simulink model "DCACmotor08022311"  (R2022b)
settings: Solver=VariableStepDiscrete  StartTime=0.0  StopTime=0.5  MaxStep=1e-4  RelTol=1e-3
libraries: spsVoltageMeasurementLib x9, spsSeriesRLCBranchLib x3, spsGroundLib x2, spsDCVoltageSourceLib x1, spsAsynchronousMachinepuUnitsLib x1, spsOnDelayLib x1, simulink x1, spsThreePhaseProgrammableVoltageSourceLib x1, spsUniversalBridgeLib x1, spsCurrentMeasurementLib x1, spspowerguiLib x1
settings Model: Creator=Lenovo  LastModifiedBy=ASUS
settings SolverCC: AlgebraicLoopSolver=TrustRegion
settings DataIOCC: ReturnWorkspaceOutputs=off
settings DebuggingCC: UnconnectedInputMsg=warning  UnconnectedOutputMsg=warning  UnconnectedLineMsg=warning  SFMachineParentedDataDiag=warning  ArithmeticOperatorsInVariantConditions=warning
settings ModelReferenceCC: EnableRefExpFcnMdlSchedulingChecks=on
settings SFSimCC: SimUseLocalCustomCode=off  CustomCodeUndefinedFunction=UseInterfaceOnly
settings RTWCC: RTWUseLocalCustomCode=off  DLArmComputeVersion=19.05

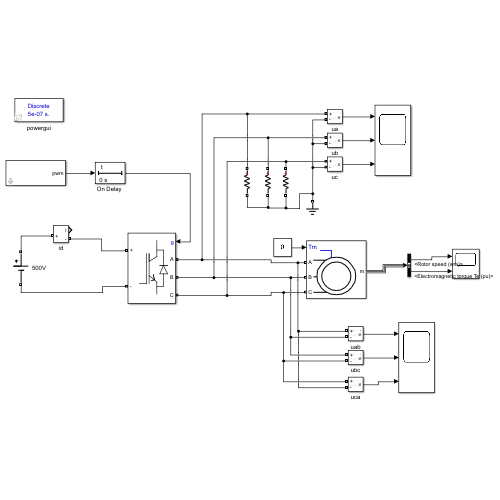
[thumbnail: Simulink's stored preview of the top-level diagram]
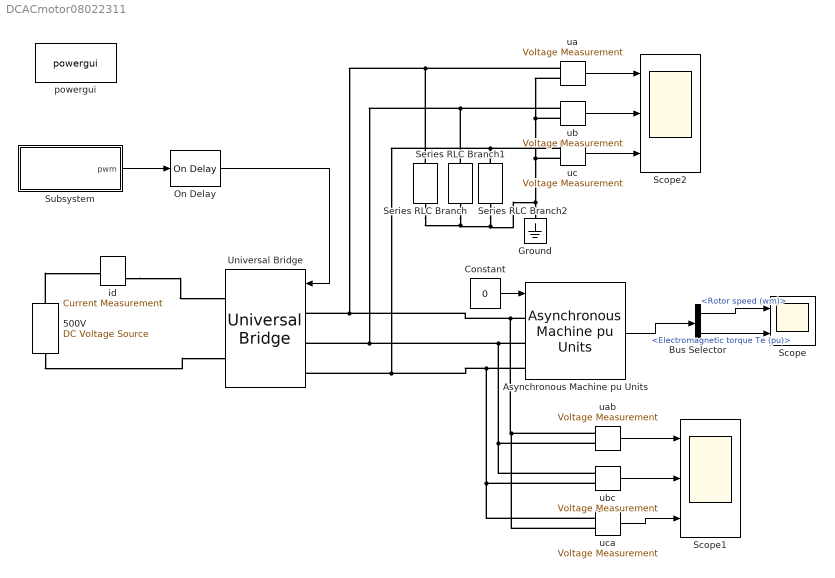
== system DCACmotor08022311 ==
  500V : spsDCVoltageSourceLib/DC Voltage Source  Amplitude=500  Measurements=None
  Asynchronous Machine pu Units : spsAsynchronousMachinepuUnitsLib/Asynchronous Machine pu Units  RotorType=Squirrel-cage  PresetModel=No  MechanicalLoad=Torque Tm  ShowDetailedParameters=on  ReferenceFrame=Rotor  Units=pu  MeasurementBus=off  NominalParameters=[3730 460 60]  VoltageRatio=1  Stator=[0.01965 0.0397]  Rotor=[0.01909 0.0397]  Cage1=[0.01909 0.0397]  Cage2=[0.01909 0.0397]  Lm=1.354  Mechanical=[0.09526 0.05479 2]  PolePairs=2  InitialConditions="[ 1,0   0,0,0   0,0,0 ]"  SimulateSaturation=off  Saturation="[0.212,0.4201,0.8125,1.0979,1.4799,2.2457,3.2586,4.5763,6.4763 ;   0.5,0.7,0.9,1,1.1,1.2 ,1.3,1.4,1.5]"  LoadFlowParameters=0  TsPowergui=0  TsBlock=-1  IterativeModel=Trapezoidal non iterative  IterativeDiscreteModel=Trapezoidal non iterative  Pmec=0
      settings: LibrarySourceBlock=|
      | sps_lib/Electrical Machines/Asynchronous Machine
      | pu Units
  Bus Selector : BusSelector  OutputSignals=Mechanical.Rotor speed (wm),Mechanical.Electromagnetic torque Te (pu)
  Constant : Constant  Value=0
  Ground : spsGroundLib/Ground  LConnTagsString=a
  "On Delay " : spsOnDelayLib/On Delay  DelayType=On delay  delay=0  ic=0  Ts=0
  Scope : Scope  NumInputPorts=2
  Scope1 : Scope  NumInputPorts=3
  Scope2 : Scope  NumInputPorts=3
  Series RLC Branch : spsSeriesRLCBranchLib/Series RLC Branch  LConnTagsString=__new0  RConnTagsString=__new0  BranchType=R  Resistance=1  Inductance=1e-3  SetiL0=off  InitialCurrent=0  Capacitance=1e-6  Setx0=off  InitialVoltage=0  Measurements=None
  Series RLC Branch1 : spsSeriesRLCBranchLib/Series RLC Branch  LConnTagsString=__new0  RConnTagsString=__new0  BranchType=R  Resistance=1  Inductance=1e-3  SetiL0=off  InitialCurrent=0  Capacitance=1e-6  Setx0=off  InitialVoltage=0  Measurements=None
  Series RLC Branch2 : spsSeriesRLCBranchLib/Series RLC Branch  LConnTagsString=__new0  RConnTagsString=__new0  BranchType=R  Resistance=1  Inductance=1e-3  SetiL0=off  InitialCurrent=0  Capacitance=1e-6  Setx0=off  InitialVoltage=0  Measurements=None
  Subsystem : Subsystem  mask{m=1, fc=1500, f=50}
      mask prompts: m "m(0<m<=1)"
  Universal Bridge : spsUniversalBridgeLib/Universal Bridge  Arms=3  SnubberResistance=1e5  SnubberCapacitance=inf  Device=IGBT / Diodes  Ron=1e-3  Lon=0  ForwardVoltages="[  0  0  ]"  ForwardVoltage=0  GTOparameters=[ 10e-6 , 20e-6 ]  IGBTparameters=[ 1e-6 , 2e-6 ]  Measurements=None  Measurements_2=None  converterType=Rectifier
  id : spsCurrentMeasurementLib/Current Measurement  PhasorSimulation=off  OutputType=Complex  PSBequivalent=0
  powergui : spspowerguiLib/powergui  Priority=1  SimulationMode=Discrete  SampleTime=5e-7  frequency=60  Iterations=50  frequencyindice=60  Pbase=100e6  ErrMax=1e-4  UnitsV=kV  UnitsW=MW  buscounter=0  FunctionMessages=off  echomessages=off  EnableUseOfTLC=off  CurrentSourceSwitches=off  DisableSnubberDevices=off  DisableRonSwitches=off  DisableVfSwitches=off  DisplayEquations=off  AutomaticDiscreteSolvers=off  SolverType=Tustin/Backward Euler (TBE)  Interpol=off  ExternalGateDelay=off  methode=off  Ts=100  x0status=blocks  SPID=on  SwTol=0  HookPort=off  NonlinearTolerance=1e-4  nMaxIteration=100  ContinueOnMaxIteration=off  RestoreLinks=warning  ResistiveCurrentMeasurement=off  Frange=[0:2:500]  Ylog=off  Xlog=on  ShowGrid=off  save=off  variable=ZData  structure=0  ZoomFFT=off  StartTime=0.0  cycles=1  DisplayStyle=1  fundamental=60  FreqAxis=off  MaxFrequency=1000  frequencyindicesteady=1  RmsSteady=1  display=off
  ua : spsVoltageMeasurementLib/Voltage Measurement  PhasorSimulation=off  OutputType=Complex  PSBequivalent=0
  uab : spsVoltageMeasurementLib/Voltage Measurement  PhasorSimulation=off  OutputType=Complex  PSBequivalent=0
  ub : spsVoltageMeasurementLib/Voltage Measurement  PhasorSimulation=off  OutputType=Complex  PSBequivalent=0
  ubc : spsVoltageMeasurementLib/Voltage Measurement  PhasorSimulation=off  OutputType=Complex  PSBequivalent=0
  uc : spsVoltageMeasurementLib/Voltage Measurement  PhasorSimulation=off  OutputType=Complex  PSBequivalent=0
  uca : spsVoltageMeasurementLib/Voltage Measurement  PhasorSimulation=off  OutputType=Complex  PSBequivalent=0
  wires:
  Subsystem/1(pwm) -> "On Delay "/1
  "On Delay "/1 -> Universal Bridge/1
  Asynchronous Machine pu Units/1 -> Bus Selector/1
  Bus Selector/2 -> Scope/2  "<Electromagnetic torque Te (pu)>"
  Bus Selector/1 -> Scope/1  "<Rotor speed (wm)>"
  Constant/1 -> Asynchronous Machine pu Units/1
  uab/1 -> Scope1/1
  ubc/1 -> Scope1/2
  uca/1 -> Scope1/3
  ub/1 -> Scope2/2
  uc/1 -> Scope2/3
  ua/1 -> Scope2/1
  connections:
  500V/LConn1 -- Universal Bridge/RConn2
  500V/RConn1 -- id/LConn1
  id/RConn1 -- Universal Bridge/RConn1
  Asynchronous Machine pu Units/LConn1 -- uca/LConn2 -- uab/LConn1 -- ua/LConn1 -- Series RLC Branch/LConn1 -- Universal Bridge/LConn1
  uab/LConn2 -- ubc/LConn1 -- Asynchronous Machine pu Units/LConn2 -- Series RLC Branch1/LConn1 -- ub/LConn1 -- Universal Bridge/LConn2
  uca/LConn1 -- ubc/LConn2 -- Asynchronous Machine pu Units/LConn3 -- Series RLC Branch2/LConn1 -- uc/LConn1 -- Universal Bridge/LConn3
  uc/LConn2 -- ua/LConn2 -- ub/LConn2 -- Series RLC Branch/RConn1 -- Series RLC Branch1/RConn1 -- Series RLC Branch2/RConn1 -- Ground/LConn1

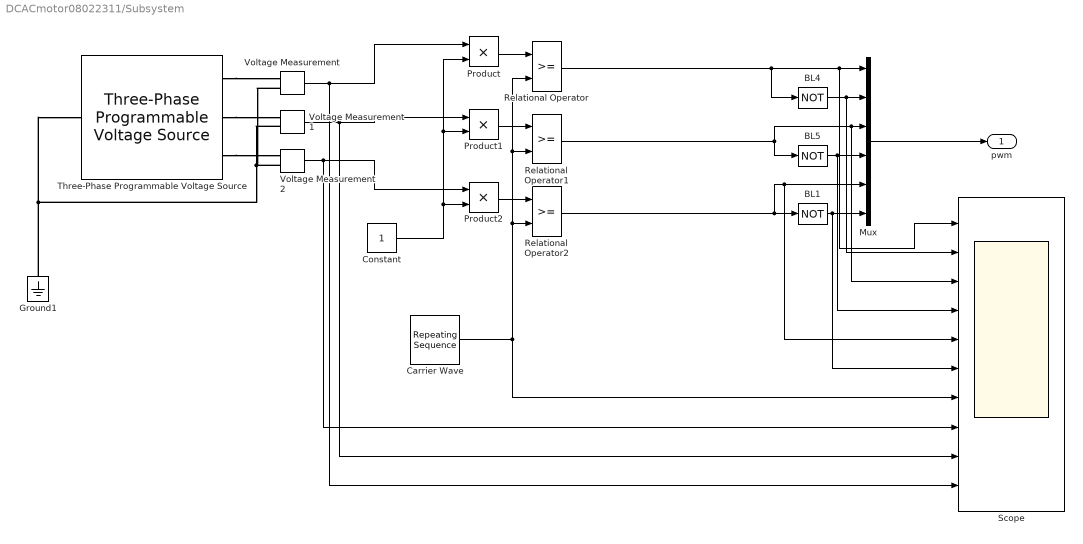
== system DCACmotor08022311/Subsystem ==
  BL1 : Logic  Operator=NOT  Inputs=1
  BL4 : Logic  Operator=NOT  Inputs=1
  BL5 : Logic  Operator=NOT  Inputs=1
  Carrier Wave : simulink/Sources/Repeating Sequence  rep_seq_t=[0 0.25/500 0.5/500 0.75/500 1/500]  rep_seq_y=[0 -1 0 1 0]
  Constant : Constant
  Ground1 : spsGroundLib/Ground  LConnTagsString=a
  Mux : Mux  Inputs=6
  Product : Product
  Product1 : Product
  Product2 : Product
  Relational Operator : RelationalOperator
  Relational Operator1 : RelationalOperator
  Relational Operator2 : RelationalOperator
  Scope : Scope  NumInputPorts=10
  Three-Phase Programmable Voltage Source : spsThreePhaseProgrammableVoltageSourceLib/Three-Phase Programmable Voltage Source  PositiveSequence="[1  0 50]"  VariationEntity=None  VariationType=Table of time-amplitude pairs  VariationTypeAlt=Step  VariationStep=0.5  VariationRate=10  VariationMagnitude=0.3  VariationFrequency=2  VariationTiming=[1 2]  VariationPhaseA=off  Amplitudes=[1 0.8 1.2 1.0]  TimeValues=[0 0.1 0.15 0.2]  HarmonicGeneration=off  HarmonicA=[3 0.2 -25 0]  HarmonicB=[2 0.15 35 2]  Timing="[0.05  3]"  BusType=swing  Pref=0  Qref=0  Qmin=-inf  Qmax=inf
  Voltage Measurement : spsVoltageMeasurementLib/Voltage Measurement  PhasorSimulation=off  OutputType=Complex  PSBequivalent=0
  Voltage Measurement1 : spsVoltageMeasurementLib/Voltage Measurement  PhasorSimulation=off  OutputType=Complex  PSBequivalent=0
  Voltage Measurement2 : spsVoltageMeasurementLib/Voltage Measurement  PhasorSimulation=off  OutputType=Complex  PSBequivalent=0
  pwm : Outport  VectorParamsAs1DForOutWhenUnconnected=off
  wires:
  Constant/1 -> Product2/2, Product1/2, Product/2
  BL1/1 -> Mux/6, Scope/6
  Relational Operator1/1 -> BL5/1, Scope/3, Mux/3
  Product/1 -> Relational Operator/1
  Mux/1 -> pwm/1
  Carrier Wave/1 -> Scope/7, Relational Operator1/2, Relational Operator/2, Relational Operator2/2
  BL5/1 -> Scope/4, Mux/4
  Product1/1 -> Relational Operator1/1
  Voltage Measurement/1 -> Scope/10, Product/1
  Relational Operator/1 -> Scope/1, Mux/1, BL4/1
  Relational Operator2/1 -> Scope/5, Mux/5, BL1/1
  BL4/1 -> Scope/2, Mux/2
  Product2/1 -> Relational Operator2/1
  Voltage Measurement2/1 -> Scope/8, Product2/1
  Voltage Measurement1/1 -> Scope/9, Product1/1
  connections:
  Ground1/LConn1 -- Voltage Measurement/LConn2 -- Voltage Measurement1/LConn2 -- Voltage Measurement2/LConn2 -- Three-Phase Programmable Voltage Source/LConn1
  Three-Phase Programmable Voltage Source/RConn1 -- Voltage Measurement/LConn1
  Three-Phase Programmable Voltage Source/RConn2 -- Voltage Measurement1/LConn1
  Three-Phase Programmable Voltage Source/RConn3 -- Voltage Measurement2/LConn1
